simulink model "TestHinfControl2States"  (R2020b)
settings: Solver=VariableStepAuto  StartTime=0.0  StopTime=50  MaxStep=0.01  RelTol=1e-3
undefined symbols (not defined in the file): a, b, Cd, K, k6, KStatic, M
libraries: simulink x1
settings Model: Creator=jeremie  LastModifiedBy=jeremie
settings DebuggingCC: ArithmeticOperatorsInVariantConditions=warning
settings SFSimCC: CustomCodeUndefinedFunction=UseInterfaceOnly

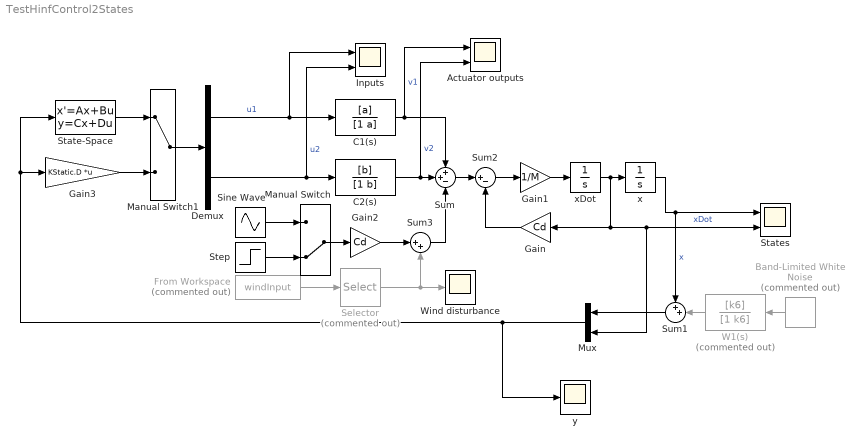
== system TestHinfControl2States ==
  Actuator outputs : Scope  NumInputPorts=2
  Band-Limited White Noise : simulink/Sources/Band-Limited White Noise  Commented=on  Cov=[0.0001]  Ts=2*pi/500  seed=[23341]
  C1(s) : TransferFcn  Numerator=[a]  Denominator=[1 a]
  C2(s) : TransferFcn  Numerator=[b]  Denominator=[1 b]
  Demux : Demux  Outputs=2
  From Workspace : FromWorkspace  Commented=on  VariableName=windInput
  Gain : Gain  Gain=Cd
  Gain1 : Gain  Gain=1/M
  Gain2 : Gain  Gain=Cd
  Gain3 : Gain  Gain=KStatic.D  Multiplication=Matrix(K*u)
  Inputs : Scope  NumInputPorts=2
  Manual Switch : ManualSwitch  CurrentSetting=0
  Manual Switch1 : ManualSwitch
  Mux : Mux  Inputs=2
  Selector : Selector  Commented=on  InputPortWidth=3  IndexOptions=Index vector (dialog)  Indices=[1]  OutputSizes=1
  Sine Wave : Sin  Amplitude=3  Frequency=0.05*2*pi  SampleTime=0
  State-Space : StateSpace  A=K.A  B=K.B  C=K.C  D=K.D  InitialCondition=0
  States : Scope  NumInputPorts=2
  Step : Step  SampleTime=0
  Sum : Sum  Inputs=++-
  Sum1 : Sum  Inputs=++|
  Sum2 : Sum  Inputs=|+-
  Sum3 : Sum  Inputs=|++
  W1(s) : TransferFcn  Commented=on  Numerator=[k6]  Denominator=[1 k6]
  Wind disturbance : Scope
  x : Integrator
  xDot : Integrator
  y : Scope
  wires:
  Sum/1 -> Sum2/1
  x/1 -> Sum1/1, States/1  "x"
  W1(s)/1 -> Sum1/2
  Demux/1 -> Inputs/1, C1(s)/1  "u1"
  Band-Limited White Noise/1 -> W1(s)/1
  Mux/1 -> y/1, Gain3/1, State-Space/1
  Demux/2 -> Inputs/2, C2(s)/1  "u2"
  xDot/1 -> Gain/1, Mux/2, States/2, x/1  "xDot"
  Sum2/1 -> Gain1/1
  Gain1/1 -> xDot/1
  Gain/1 -> Sum2/2
  Manual Switch/1 -> Gain2/1
  Sum3/1 -> Sum/3
  C2(s)/1 -> Actuator outputs/2, Sum/2  "v2"
  C1(s)/1 -> Actuator outputs/1, Sum/1  "v1"
  Sine Wave/1 -> Manual Switch/1
  Step/1 -> Manual Switch/2
  Gain2/1 -> Sum3/1
  From Workspace/1 -> Selector/1
  Selector/1 -> Wind disturbance/1, Sum3/2
  Manual Switch1/1 -> Demux/1
  Gain3/1 -> Manual Switch1/2
  State-Space/1 -> Manual Switch1/1
  Sum1/1 -> Mux/1
